simulink model "Proj_4"  (R2024a)
settings: Solver=VariableStepAuto  StartTime=0.0  StopTime=10.0  RelTol=1e-3
values from neighbouring files (symbols this model uses):
  rps2rpm = 60/(2*pi())    [wk3_init.m]
undefined symbols (not defined in the file or in its folder): batData, carData, motorData
libraries: slpidlib x1
settings Model: Creator=cbvaw  LastModifiedBy=stick
settings RTWCC: GPUComputeCapability=3.5

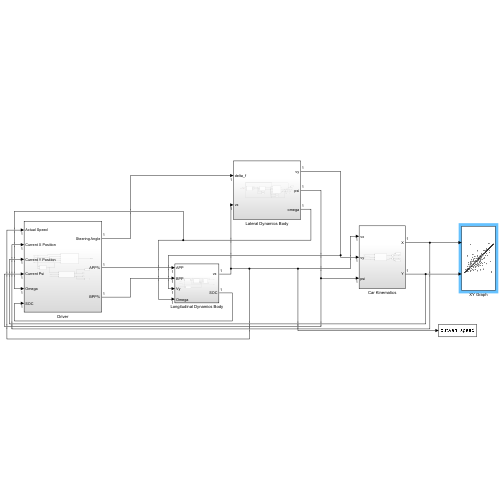
[thumbnail: Simulink's stored preview of the top-level diagram]
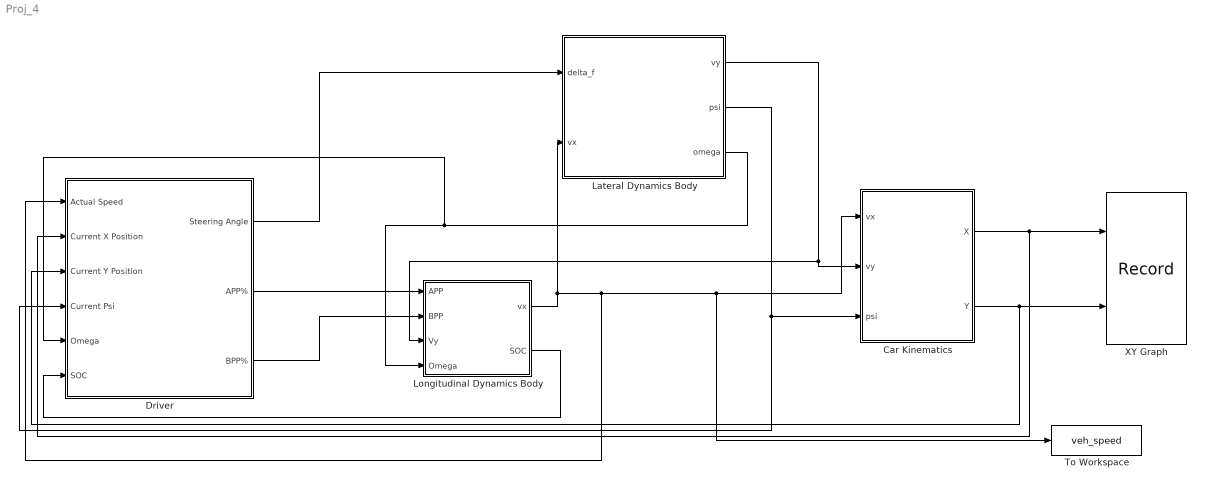
== system Proj_4 ==
  Car Kinematics : Subsystem
  Driver : Subsystem
  Lateral Dynamics Body : Subsystem
  Longitudinal Dynamics Body : Subsystem
  To Workspace : ToWorkspace  VariableName=veh_speed  SaveFormat=Structure With Time  SampleTime=-1
  XY Graph : Record  FileSettingsInternal="{\"entries\":[{\"content\":{\"excelSettings\":{\"content\":{},\"type\":\"Streamout.ExcelSettings\"}},\"type\":\"Streamout.FileSettingStorage\",\"uuid\":\"\"}],\"packageUris\":[\"http:\\/\\/schema.mathworks.com\\/mf0\\/streamout_blocks\\/R2020a\"],\"version\":\"1.0\"}"  Layout=[1 1]  SignalsInternal="{\"entries\":[{\"content\":{\"signals\":[{\"content\":{\"blockPath\":[],\"dimensions\":[1],\"domain\":\"\",\"lineColor\":\"#d95319\",\"plots\":[ 1 ],\"port\":1,\"signalID\":1,\"signalName\":\"CarKinematicsInertialFrame:1\"},\"type\":\"RecordBlkView.Signal\",\"uuid\":\"\"},{\"content\":{\"blockPath\":[],\"dimensions\":[1],\"domain\":\"\",\"lineColor\":\"#edb120\",\"plots\":[ 1 ],\"port\":2,\"signalID\":2,\"signalName\":\"CarKinematicsInertialFrame:2\"},\"type\":\"RecordBlkView.Signal\",\"uuid\":\"\"}]},\"type\":\"RecordBlkView.InputSignals\",\"uuid\":\"\"}],\"packageUris\":[\"http:\\/\\/schema.mathworks.com\\/mf0\\/streamout_blocks\\/R2020a\"],\"version\":\"1.0\"}"  VisualizationBindings="{\"xyplotplugin\":{\"info\":[{\"series\":[{\"bindingParametersList\":[{\"parameter\":\"X-Axis\",\"signalID\":1,\"signalName\":\"CarKinematicsInertialFrame:1\"},{\"parameter\":\"Y-Axis\",\"signalID\":2,\"signalName\":\"CarKinematicsInertialFrame:2\"}],\"seriesID\":0}],\"subplotID\":1}]}}"  CompatibilityTag=XY  st=-1
  wires:
  Car Kinematics/2(Y) -> Driver/3(Current Y Position), XY Graph/2
  Car Kinematics/1(X) -> Driver/2(Current X Position), XY Graph/1
  Lateral Dynamics Body/1(vy) -> Longitudinal Dynamics Body/3(Vy), Car Kinematics/2(vy)
  Lateral Dynamics Body/2(psi) -> Driver/4(Current Psi), Car Kinematics/3(psi)
  Longitudinal Dynamics Body/1("vx ") -> Driver/1(Actual Speed), To Workspace/1, Car Kinematics/1(vx), Lateral Dynamics Body/2(vx)
  Lateral Dynamics Body/3(omega) -> Driver/5(Omega), Longitudinal Dynamics Body/4(Omega)
  Driver/2(APP%) -> Longitudinal Dynamics Body/1(APP)
  Driver/3(BPP%) -> Longitudinal Dynamics Body/2(BPP)
  Driver/1(Steering Angle) -> Lateral Dynamics Body/1(delta_f)
  Longitudinal Dynamics Body/2(SOC) -> Driver/6(SOC)

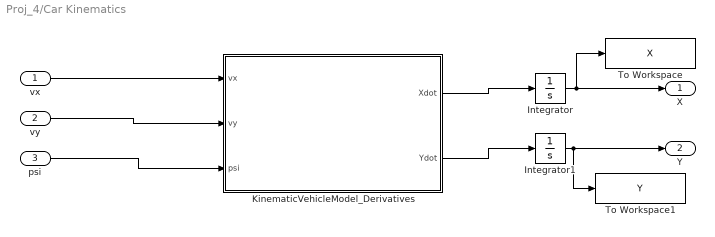
== system Proj_4/Car Kinematics ==
  vx : Inport
  vy : Inport  Port=2
  psi : Inport  Port=3
  Integrator : Integrator  InitialCondition=carData.init.X0
  Integrator1 : Integrator  InitialCondition=carData.init.Y0
  KinematicVehicleModel_Derivatives : MATLAB Function  TreatAsAtomicUnit=on
  To Workspace : ToWorkspace  VariableName=X  SaveFormat=Timeseries  SampleTime=-1
  To Workspace1 : ToWorkspace  VariableName=Y  SaveFormat=Timeseries  SampleTime=-1
  X : Outport
  Y : Outport  Port=2
  wires:
  Integrator1/1 -> To Workspace1/1, Y/1
  vy/1 -> KinematicVehicleModel_Derivatives/2(vy)
  vx/1 -> KinematicVehicleModel_Derivatives/1(vx)
  KinematicVehicleModel_Derivatives/2(Ydot) -> Integrator1/1
  psi/1 -> KinematicVehicleModel_Derivatives/3(psi)
  Integrator/1 -> To Workspace/1, X/1
  KinematicVehicleModel_Derivatives/1(Xdot) -> Integrator/1

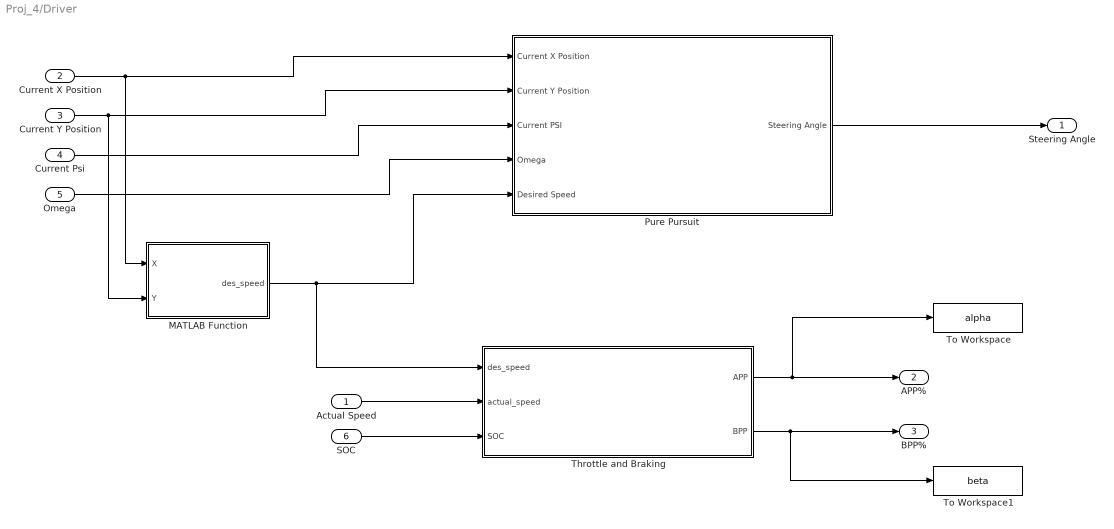
== system Proj_4/Driver ==
  Actual Speed : Inport
  Current X Position : Inport  Port=2
  Current Y Position : Inport  Port=3
  Current Psi : Inport  Port=4
  Omega : Inport  Port=5
  SOC : Inport  Port=6
  MATLAB Function : MATLAB Function  TreatAsAtomicUnit=on
  Pure Pursuit : Subsystem
  Throttle and Braking : Subsystem
  To Workspace : ToWorkspace  VariableName=alpha  SaveFormat=Timeseries  SampleTime=-1
  To Workspace1 : ToWorkspace  VariableName=beta  SaveFormat=Timeseries  SampleTime=-1
  Steering Angle : Outport
  APP% : Outport  Port=2
  BPP% : Outport  Port=3
  wires:
  Throttle and Braking/2(BPP) -> BPP%/1, To Workspace1/1
  Throttle and Braking/1(APP) -> APP%/1, To Workspace/1
  SOC/1 -> Throttle and Braking/3(SOC)
  Actual Speed/1 -> Throttle and Braking/2(actual_speed)
  Pure Pursuit/1(Steering Angle) -> Steering Angle/1
  MATLAB Function/1(des_speed) -> Pure Pursuit/5(Desired Speed), Throttle and Braking/1(des_speed)
  Omega/1 -> Pure Pursuit/4(Omega)
  Current Psi/1 -> Pure Pursuit/3(Current PSI)
  Current Y Position/1 -> MATLAB Function/2(Y), Pure Pursuit/2(Current Y Position)
  Current X Position/1 -> MATLAB Function/1(X), Pure Pursuit/1(Current X Position)

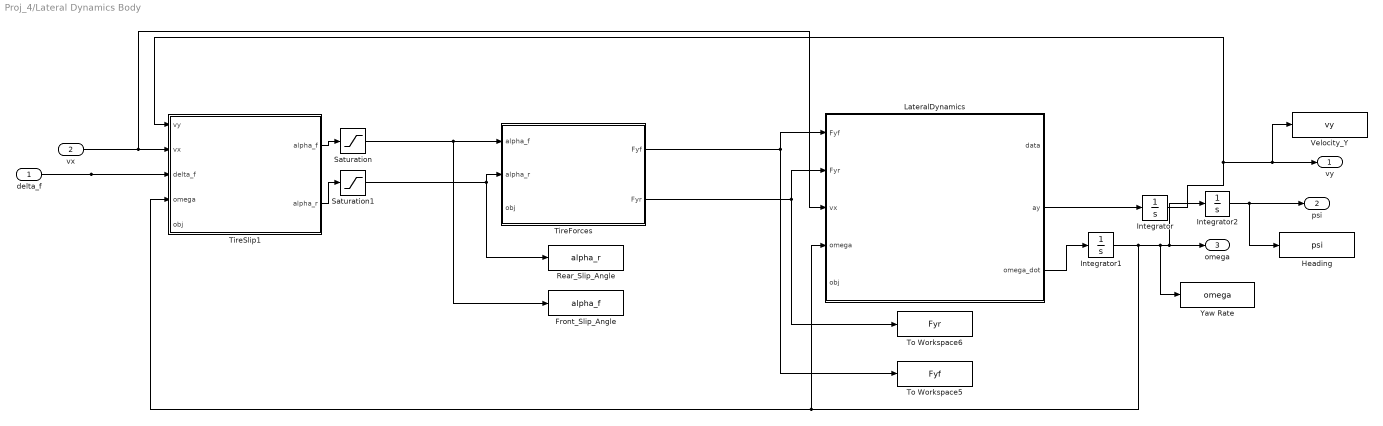
== system Proj_4/Lateral Dynamics Body ==
  delta_f : Inport
  vx : Inport  Port=2
  Front_Slip_Angle : ToWorkspace  VariableName=alpha_f  SaveFormat=Timeseries  SampleTime=-1
  Heading : ToWorkspace  VariableName=psi  SaveFormat=Timeseries  SampleTime=-1
  Integrator : Integrator  InitialCondition=carData.init.vy0
  Integrator1 : Integrator  InitialCondition=carData.init.omega0
  Integrator2 : Integrator  InitialCondition=carData.init.psi0  WrappedStateUpperValue=2*pi  WrappedStateLowerValue=0
  LateralDynamics : MATLAB Function  TreatAsAtomicUnit=on
  Rear_Slip_Angle : ToWorkspace  VariableName=alpha_r  SaveFormat=Timeseries  SampleTime=-1
  Saturation : Saturate  UpperLimit=carData.maxAlpha  LowerLimit=-carData.maxAlpha
  Saturation1 : Saturate  UpperLimit=carData.maxAlpha  LowerLimit=-carData.maxAlpha
  TireForces : MATLAB Function  TreatAsAtomicUnit=on
  TireSlip1 : MATLAB Function  TreatAsAtomicUnit=on
  To Workspace5 : ToWorkspace  VariableName=Fyf  SaveFormat=Timeseries  SampleTime=-1
  To Workspace6 : ToWorkspace  VariableName=Fyr  SaveFormat=Timeseries  SampleTime=-1
  Velocity_Y : ToWorkspace  VariableName=vy  SaveFormat=Timeseries  SampleTime=-1
  Yaw Rate : ToWorkspace  VariableName=omega  SaveFormat=Timeseries  SampleTime=-1
  vy : Outport
  psi : Outport  Port=2
  omega : Outport  Port=3
  wires:
  Integrator1/1 -> Integrator2/1, omega/1, Yaw Rate/1, LateralDynamics/4(omega), TireSlip1/4(omega)
  delta_f/1 -> TireSlip1/3(delta_f)
  Integrator/1 -> TireSlip1/1(vy), vy/1, Velocity_Y/1
  LateralDynamics/3(omega_dot) -> Integrator1/1
  Integrator2/1 -> Heading/1, psi/1
  LateralDynamics/2(ay) -> Integrator/1
  Saturation1/1 -> TireForces/2(alpha_r), Rear_Slip_Angle/1
  TireSlip1/1(alpha_f) -> Saturation/1
  vx/1 -> LateralDynamics/3(vx), TireSlip1/2(vx)
  TireForces/2(Fyr) -> LateralDynamics/2(Fyr), To Workspace6/1
  TireForces/1(Fyf) -> LateralDynamics/1(Fyf), To Workspace5/1
  Saturation/1 -> TireForces/1(alpha_f), Front_Slip_Angle/1
  TireSlip1/2(alpha_r) -> Saturation1/1

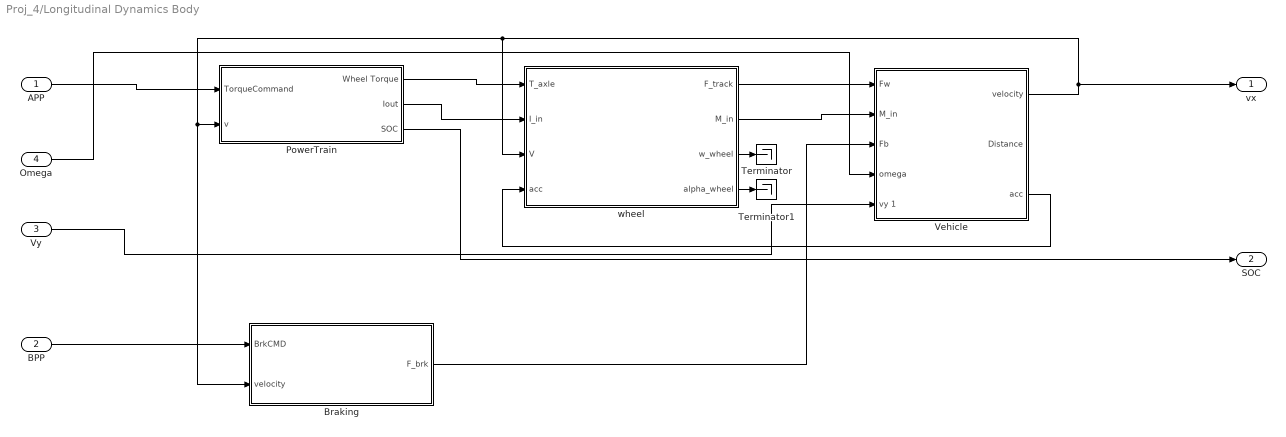
== system Proj_4/Longitudinal Dynamics Body ==
  APP : Inport
  BPP : Inport  Port=2
  Vy : Inport  Port=3
  Omega : Inport  Port=4
  Braking : Subsystem
  PowerTrain : Subsystem
  Terminator : Terminator
  Terminator1 : Terminator
  Vehicle : Subsystem
  "wheel " : Subsystem
  "vx " : Outport
  SOC : Outport  Port=2
  wires:
  PowerTrain/1(Wheel Torque) -> "wheel "/1(T_axle)
  PowerTrain/2(Iout) -> "wheel "/2(I_in)
  Braking/1("F_brk ") -> Vehicle/3("Fb ")
  "wheel "/2(M_in) -> Vehicle/2("M_in ")
  "wheel "/1(F_track) -> Vehicle/1("Fw ")
  Vehicle/1("velocity ") -> Braking/2("velocity "), PowerTrain/2(v), "wheel "/3(V), "vx "/1
  Vehicle/3(acc) -> "wheel "/4(acc)
  APP/1 -> PowerTrain/1(TorqueCommand)
  BPP/1 -> Braking/1("BrkCMD ")
  PowerTrain/3(SOC) -> SOC/1
  Vy/1 -> Vehicle/5(vy 1)
  Omega/1 -> Vehicle/4(omega)
  "wheel "/3(w_wheel) -> Terminator/1
  "wheel "/4(alpha_wheel) -> Terminator1/1

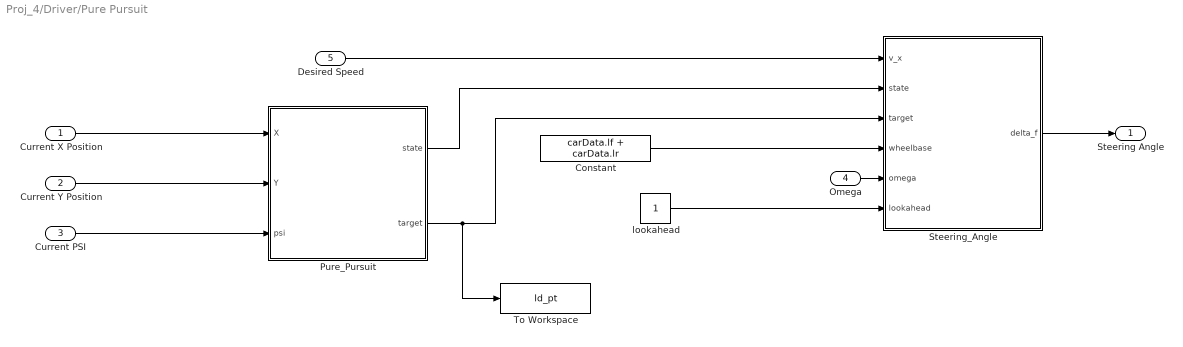
== system Proj_4/Driver/Pure Pursuit ==
  Current X Position : Inport
  Current Y Position : Inport  Port=2
  Current PSI : Inport  Port=3
  Omega : Inport  Port=4
  Desired Speed : Inport  Port=5
  Constant : Constant  Value=carData.lf + carData.lr
  Pure_Pursuit : MATLAB Function  TreatAsAtomicUnit=on
  Steering_Angle : MATLAB Function  TreatAsAtomicUnit=on
  To Workspace : ToWorkspace  VariableName=ld_pt  SaveFormat=Timeseries  SampleTime=-1
  lookahead : Constant
  Steering Angle : Outport
  wires:
  Constant/1 -> Steering_Angle/4(wheelbase)
  lookahead/1 -> Steering_Angle/6(lookahead)
  Steering_Angle/1(delta_f) -> Steering Angle/1
  Pure_Pursuit/2(target) -> Steering_Angle/3(target), To Workspace/1
  Omega/1 -> Steering_Angle/5(omega)
  Pure_Pursuit/1(state) -> Steering_Angle/2(state)
  Desired Speed/1 -> Steering_Angle/1(v_x)
  Current PSI/1 -> Pure_Pursuit/3(psi)
  Current Y Position/1 -> Pure_Pursuit/2(Y)
  Current X Position/1 -> Pure_Pursuit/1(X)

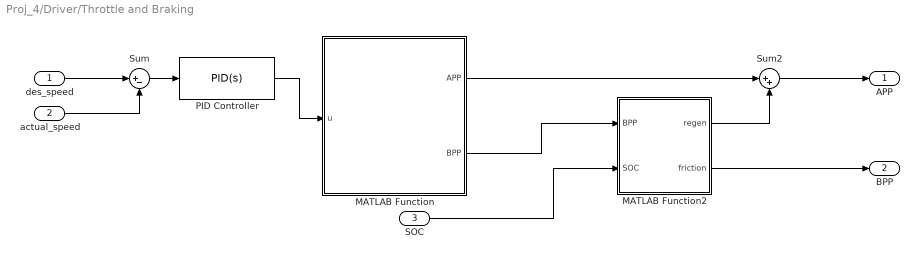
== system Proj_4/Driver/Throttle and Braking ==
  des_speed : Inport
  actual_speed : Inport  Port=2
  SOC : Inport  Port=3
  MATLAB Function : MATLAB Function  TreatAsAtomicUnit=on
  MATLAB Function2 : MATLAB Function  TreatAsAtomicUnit=on
  PID Controller : slpidlib/PID Controller  Controller=PID  Form=Parallel  TimeDomain=Continuous-time  UseExternalTs=off  SampleTime=-1  IntegratorMethod=Forward Euler  FilterMethod=Forward Euler  ControllerParametersSource=internal  P=.6  I=0  UseKiTs=off  D=.001  UseExternalDerivativeSource=off  N=100  UseFilter=on  TunerSelectOption=Transfer Function Based (PID Tuner App)  InitialConditionSource=internal  InitialConditionForIntegrator=0  InitialConditionForFilter=0  DifferentiatorICPrevScaledInput=0  ExternalReset=none  TrackingMode=off  Kt=1  LimitOutput=on  SatLimitsSource=internal  UpperSaturationLimit=1  LowerSaturationLimit=-1  LinearizeAsGain=off  AntiWindupMode=none  Kb=1  LimitIntegrator=off  UpperIntegratorSaturationLimit=inf  LowerIntegratorSaturationLimit=-inf  POutMin=[]  POutMax=[]  IOutMin=[]  IOutMax=[]  DOutMin=[]  DOutMax=[]  NOutMin=[]  NOutMax=[]  SumOutMin=[]  SumOutMax=[]  SaturationOutMin=[]  SaturationOutMax=[]  PParamMin=[]  PParamMax=[]  IParamMin=[]  IParamMax=[]  DParamMin=[]  DParamMax=[]  NParamMin=[]  NParamMax=[]  KbParamMin=[]  KbParamMax=[]  KtParamMin=[]  KtParamMax=[]  KbOutMin=[]  KbOutMax=[]  KtOutMin=[]  KtOutMax=[]  IntegratorOutMin=[]  IntegratorOutMax=[]  FilterOutMin=[]  FilterOutMax=[]  SumI1OutMin=[]  SumI1OutMax=[]  SumI2OutMin=[]  SumI2OutMax=[]  SumI3OutMin=[]  SumI3OutMax=[]  SumI4OutMin=[]  SumI4OutMax=[]  SumDOutMin=[]  SumDOutMax=[]  DifferentiatorOutMin=[]  DifferentiatorOutMax=[]  FilterDiffOutCoefMin=[]  FilterDiffOutCoefMax=[]  ReciprocalOutMin=[]  ReciprocalOutMax=[]  SumDenOutMin=[]  SumDenOutMax=[]  SumNumOutMin=[]  SumNumOutMax=[]  DivideOutMin=[]  DivideOutMax=[]  UdiffTsProdOutMin=[]  UdiffTsProdOutMax=[]  NTsProdOutMin=[]  NTsProdOutMax=[]  UintegralTsProdOutMin=[]  UintegralTsProdOutMax=[]  UngainTsProdOutMin=[]  UngainTsProdOutMax=[]  ClampingZeroOutDataTypeStr=Inherit: Inherit via back propagation  ClampingZeroOutMin=[]  ClampingZeroOutMax=[]  FilterDenConstantOutDataTypeStr=Inherit: Inherit via back propagation  FilterDenConstantOutMin=[]  FilterDenConstantOutMax=[]  PCopyOutDataTypeStr=Inherit: Inherit via back propagation  PCopyOutMin=[]  PCopyOutMax=[]  NCopyOutDataTypeStr=Inherit: Inherit via back propagation  NCopyOutMin=[]  NCopyOutMax=[]  IntegratorContinuousStateAttributes=''  IntegratorStateMustResolveToSignalObject=off  IntegratorRTWStateStorageClass=Auto  FilterContinuousStateAttributes=''  FilterStateMustResolveToSignalObject=off  FilterRTWStateStorageClass=Auto  ParallelPVariant=InternalParameters  IdealPVariant=Disabled  IVariant=InternalParameters  DVariant=InternalParameters  IntegratorVariant=Continuous  SatVariant=Enabled  AWVariant=Passthrough  PCopyVariant=Disabled  TRVariant=Disabled  FdbkBlocksVariant=Forward  IdealPFdbkVariant=Disabled  SatFdbkVariant=Disabled  DerivativeFilterVariant=ContFilter  NVariant=InternalParameters  NCopyVariant=Disabled  FilterICVariant=InternalICsFilter  IntegratorICVariant=InternalICs  ExternalResetVariant=Disabled  TRSumVariant=Passthrough  SumFdbkVariant=Disabled  SumVariant=Sum_PID  TsampFilterVariant=InternalTs  TsampNgainVariant=Passthrough  TsampIntegralVariant=Disabled_SignalSpec  ExternalSaturationOutDataTypeStr=Inherit: Same as second input  DerivativeSourceVariant=ErrorSignal
  Sum : Sum  Inputs=|+-
  Sum2 : Sum  Inputs=|++
  APP : Outport
  BPP : Outport  Port=2
  wires:
  MATLAB Function2/2(friction) -> BPP/1
  Sum2/1 -> APP/1
  MATLAB Function2/1(regen) -> Sum2/2
  PID Controller/1 -> MATLAB Function/1(u)
  Sum/1 -> PID Controller/1
  MATLAB Function/2(BPP) -> MATLAB Function2/1(BPP)
  MATLAB Function/1(APP) -> Sum2/1
  SOC/1 -> MATLAB Function2/2(SOC)
  actual_speed/1 -> Sum/2
  des_speed/1 -> Sum/1

== system Proj_4/Longitudinal Dynamics Body/Braking ==
  "BrkCMD " : Inport
  "velocity " : Inport  Port=2
  Gain1 : Gain  Gain=10000*carData.r
  MATLAB Function : MATLAB Function  TreatAsAtomicUnit=on
  "F_brk " : Outport  VectorParamsAs1DForOutWhenUnconnected=off
  wires:
  "BrkCMD "/1 -> Gain1/1
  Gain1/1 -> MATLAB Function/1(u)
  MATLAB Function/1(y) -> "F_brk "/1
  "velocity "/1 -> MATLAB Function/2(v)

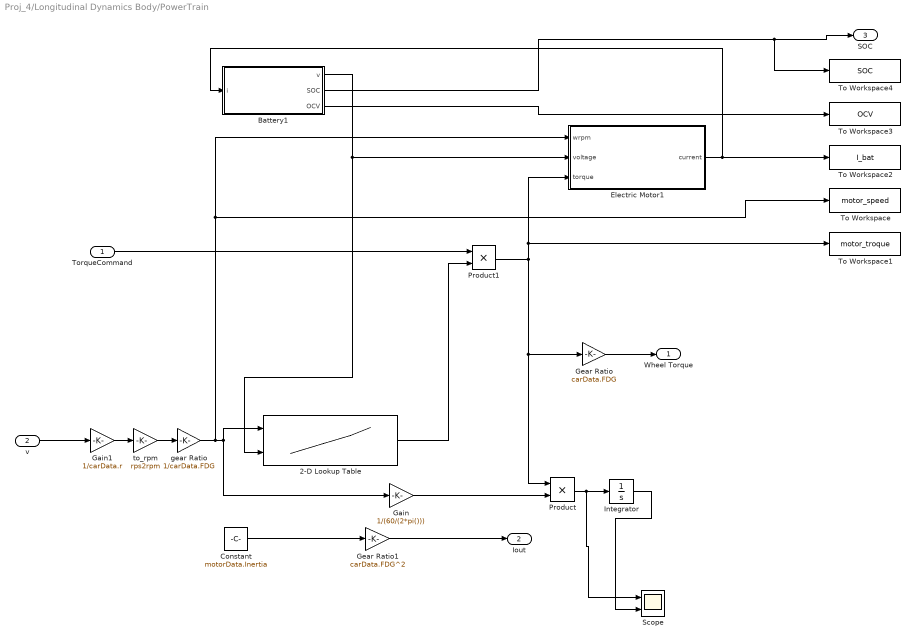
== system Proj_4/Longitudinal Dynamics Body/PowerTrain ==
  TorqueCommand : Inport
  v : Inport  Port=2
  2-D Lookup Table : Lookup_n-D  BreakpointsForDimension1=motorData.vbus  BreakpointsForDimension2=motorData.rpm  Table=motorData.maxtorque  InternalRulePriority=Speed  RndMeth=Simplest
      settings: InputPortMap=u0,u1
  Battery1 : Subsystem
  Constant : Constant  Value=motorData.Inertia
  Electric Motor1 : Subsystem
  Gain : Gain  Gain=1/(60/(2*pi()))
  Gain1 : Gain  Gain=1/carData.r
  Gear Ratio : Gain  Gain=carData.FDG
  Gear Ratio1 : Gain  Gain=carData.FDG^2
  Integrator : Integrator
  Product : Product
  Product1 : Product
  Scope : Scope  NumInputPorts=2
  To Workspace : ToWorkspace  VariableName=motor_speed  SaveFormat=Structure With Time  SampleTime=-1
  To Workspace1 : ToWorkspace  VariableName=motor_troque  SaveFormat=Structure With Time  SampleTime=-1
  To Workspace2 : ToWorkspace  VariableName=I_bat  SaveFormat=Structure With Time  SampleTime=-1
  To Workspace3 : ToWorkspace  VariableName=OCV  SaveFormat=Structure With Time  SampleTime=-1
  To Workspace4 : ToWorkspace  VariableName=SOC  SaveFormat=Structure With Time  SampleTime=-1
  gear Ratio : Gain  Gain=1/carData.FDG
  to_rpm : Gain  Gain=rps2rpm
  Wheel Torque : Outport
  Iout : Outport  Port=2
  SOC : Outport  Port=3
  wires:
  TorqueCommand/1 -> Product1/1
  Constant/1 -> Gear Ratio1/1
  v/1 -> Gain1/1
  Gain1/1 -> to_rpm/1
  2-D Lookup Table/1 -> Product1/2
  Product1/1 -> Product/1, Gear Ratio/1, Electric Motor1/3(torque), To Workspace1/1
  to_rpm/1 -> gear Ratio/1
  gear Ratio/1 -> Electric Motor1/1(wrpm), To Workspace/1, Gain/1, 2-D Lookup Table/1
  Gear Ratio/1 -> Wheel Torque/1
  Product/1 -> Scope/1, Integrator/1
  Integrator/1 -> Scope/2
  Gain/1 -> Product/2
  Battery1/1(v) -> 2-D Lookup Table/2, Electric Motor1/2(voltage)
  Electric Motor1/1(current) -> To Workspace2/1, Battery1/1(i)
  Gear Ratio1/1 -> Iout/1
  Battery1/2(SOC) -> To Workspace4/1, SOC/1
  Battery1/3(OCV) -> To Workspace3/1

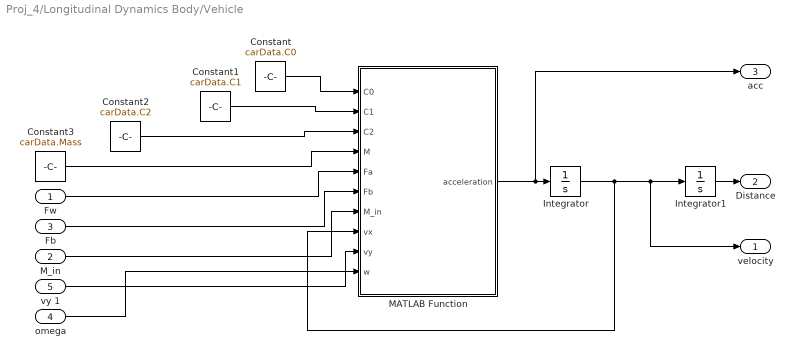
== system Proj_4/Longitudinal Dynamics Body/Vehicle ==
  "Fw " : Inport
  "M_in " : Inport  Port=2
  "Fb " : Inport  Port=3
  omega : Inport  Port=4
  vy 1 : Inport  Port=5
  Constant : Constant  Value=carData.C0
  Constant1 : Constant  Value=carData.C1
  Constant2 : Constant  Value=carData.C2
  Constant3 : Constant  Value=carData.Mass
  Integrator : Integrator  LimitOutput=on  LowerSaturationLimit=0
  Integrator1 : Integrator
  MATLAB Function : MATLAB Function  TreatAsAtomicUnit=on
  "velocity " : Outport  VectorParamsAs1DForOutWhenUnconnected=off
  "Distance " : Outport  Port=2  VectorParamsAs1DForOutWhenUnconnected=off
  acc : Outport  Port=3
  wires:
  Constant1/1 -> MATLAB Function/2(C1)
  Constant/1 -> MATLAB Function/1(C0)
  MATLAB Function/1(acceleration) -> acc/1, Integrator/1
  Constant2/1 -> MATLAB Function/3(C2)
  Constant3/1 -> MATLAB Function/4(M)
  "Fw "/1 -> MATLAB Function/5(Fa)
  "Fb "/1 -> MATLAB Function/6(Fb)
  Integrator/1 -> MATLAB Function/8(vx), "velocity "/1, Integrator1/1
  Integrator1/1 -> "Distance "/1
  "M_in "/1 -> MATLAB Function/7(M_in)
  omega/1 -> MATLAB Function/10(w)
  vy 1/1 -> MATLAB Function/9(vy)

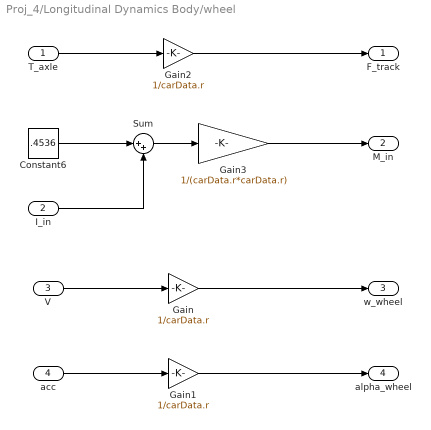
== system Proj_4/Longitudinal Dynamics Body/wheel  ==
  T_axle : Inport
  I_in : Inport  Port=2
  V : Inport  Port=3
  acc : Inport  Port=4
  Constant6 : Constant  Value=.4536
  Gain : Gain  Gain=1/carData.r
  Gain1 : Gain  Gain=1/carData.r
  Gain2 : Gain  Gain=1/carData.r
  Gain3 : Gain  Gain=1/(carData.r*carData.r)
  Sum : Sum  Inputs=|++
  F_track : Outport
  M_in : Outport  Port=2
  w_wheel : Outport  Port=3
  alpha_wheel : Outport  Port=4
  wires:
  Gain/1 -> w_wheel/1
  V/1 -> Gain/1
  acc/1 -> Gain1/1
  Gain1/1 -> alpha_wheel/1
  T_axle/1 -> Gain2/1
  Gain2/1 -> F_track/1
  Gain3/1 -> M_in/1
  Constant6/1 -> Sum/1
  I_in/1 -> Sum/2
  Sum/1 -> Gain3/1

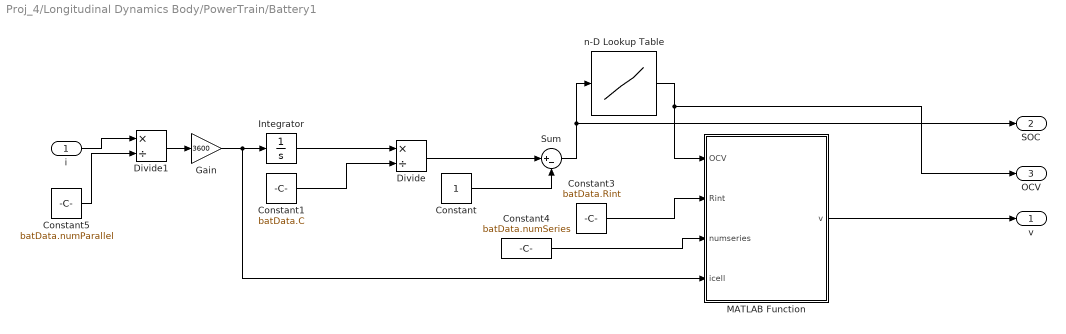
== system Proj_4/Longitudinal Dynamics Body/PowerTrain/Battery1 ==
  i : Inport
  Constant : Constant
  Constant1 : Constant  Value=batData.C
  Constant3 : Constant  Value=batData.Rint
  Constant4 : Constant  Value=batData.numSeries
  Constant5 : Constant  Value=batData.numParallel
  Divide : Product  Inputs=*/
  Divide1 : Product  Inputs=*/
  Gain : Gain  Gain=3600
  Integrator : Integrator
  MATLAB Function : MATLAB Function  TreatAsAtomicUnit=on
  Sum : Sum  Inputs=|+-
  n-D Lookup Table : Lookup_n-D  NumberOfTableDimensions=1  BreakpointsForDimension1=batData.SOC  BreakpointsForDimension3=[5, 7]  Table=batData.OCV  InternalRulePriority=Speed  RndMeth=Simplest
  v : Outport
  SOC : Outport  Port=2
  OCV : Outport  Port=3
  wires:
  Constant/1 -> Sum/2
  Integrator/1 -> Divide/1
  Divide/1 -> Sum/1
  Constant1/1 -> Divide/2
  MATLAB Function/1(v) -> v/1
  Constant4/1 -> MATLAB Function/3(numseries)
  Divide1/1 -> Gain/1
  Constant5/1 -> Divide1/2
  i/1 -> Divide1/1
  Constant3/1 -> MATLAB Function/2(Rint)
  Sum/1 -> SOC/1, n-D Lookup Table/1
  n-D Lookup Table/1 -> OCV/1, MATLAB Function/1(OCV)
  Gain/1 -> MATLAB Function/4(icell), Integrator/1

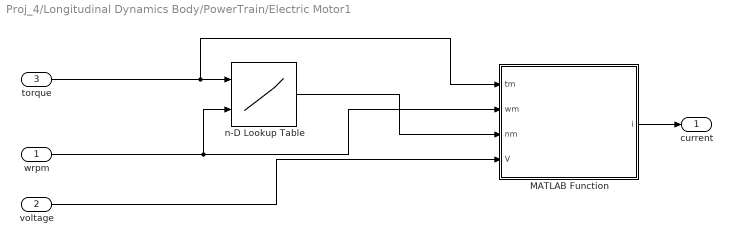
== system Proj_4/Longitudinal Dynamics Body/PowerTrain/Electric Motor1 ==
  wrpm : Inport
  voltage : Inport  Port=2
  torque : Inport  Port=3
  MATLAB Function : MATLAB Function  TreatAsAtomicUnit=on
  n-D Lookup Table : Lookup_n-D  BreakpointsForDimension1=motorData.eta_torque  BreakpointsForDimension2=motorData.eta_speed  BreakpointsForDimension3=[5, 7]  Table=motorData.eta_val  InternalRulePriority=Speed  RndMeth=Simplest
      settings: InputPortMap=u0,u1
  current : Outport
  wires:
  torque/1 -> MATLAB Function/1(tm), n-D Lookup Table/1
  wrpm/1 -> MATLAB Function/2(wm), n-D Lookup Table/2
  n-D Lookup Table/1 -> MATLAB Function/3(nm)
  MATLAB Function/1(i) -> current/1
  voltage/1 -> MATLAB Function/4(V)

== matlab function Proj_4/Driver/Pure Pursuit/Pure_Pursuit ==
  data: state output; target output; X input; Y input; psi input
function [state,target] = fcn(X,Y, psi)

dist = zeros(1, numel(waypoints_x));

for i = 1:numel(waypoints_x)
    dist(i) = sqrt((waypoints_x(i) - X)^2 + (waypoints_y(i) - Y)^2);

end

[~, index] = min(dist);

target_psi = atan2(waypoints_y(index) - Y, waypoints_x(index) - X);


state =[X,Y,psi];

target = [waypoints_x(index), waypoints_y(index), target_psi];

== matlab function Proj_4/Driver/Pure Pursuit/Steering_Angle ==
  data: v_x input; delta_f output; state input; target input; wheelbase input; omega input; lookahead input
function delta_f = fcn(v_x, state, target, wheelbase, omega, lookahead)

X = state(1);
Y = state(2);
psi = state(3);

target_X = target(1)
target_Y = target(2)
target_psi = target(3)

alpha = atan2(target_Y - Y, target_X - X) - psi;
psi_dot = (2 * wheelbase * sin(alpha)) / lookahead;
delta_f = atan(psi_dot);

== matlab function Proj_4/Driver/Throttle and Braking/MATLAB Function ==
  data: APP output; u input; BPP output
function [APP,BPP] = fcn(u)

if u>0
    APP=u;
    BPP=0;
elseif u<0
    APP=0;
    BPP=-u;
else
    APP=0;
    BPP=0;
end

== matlab function Proj_4/Driver/Throttle and Braking/MATLAB Function2 ==
  data: BPP input; regen output; friction output; SOC input
function [regen, friction] = fcn(BPP,SOC)

if actual_speed < 5
    friction = BPP;
    regen = 0;

elseif actual_speed >= 5 && actual_speed <= 25
    friction = BPP * ((100 - 4.75 * (actual_speed - 5)) / 100);
    regen = (1 - ((100 - 4.75 * (actual_speed - 5)) / 100)) * BPP;

else
    friction = 0.05 * BPP;
    regen = 0.95 * BPP;

end

if SOC >= 95
    friction = BPP;
    regen = 0;
end

== matlab function Proj_4/Lateral Dynamics Body/TireSlip1 ==
  data: vy input; alpha_f output; vx input; delta_f input; omega input; obj input; alpha_r output
function [alpha_f, alpha_r] = fnc(vy, vx, delta_f, omega, obj)

    if abs(vx) > obj.vx_threshold1
        alpha_f = delta_f - (vy + omega * obj.lf) / vx;
        alpha_r = - (vy - omega * obj.lr) / vx;
    else
        alpha_f = 0;
        alpha_r = 0;
    end

end

== matlab function Proj_4/Lateral Dynamics Body/LateralDynamics ==
  data: data output; Fyf input; ay output; Fyr input; vx input; omega input; obj input; omega_dot output
function [data, ay, omega_dot] = fcn(Fyf, Fyr, vx, omega, obj)

    Fy = Fyf + Fyr;
    ay = Fy / obj.Mass - omega * vx;

    M = Fyf * obj.lf - Fyr * obj.lr;
    omega_dot = M / obj.Inertia;

end

== matlab function Proj_4/Longitudinal Dynamics Body/PowerTrain/Electric Motor1/MATLAB Function ==
  data: tm input; i output; wm input; nm input; V input
function i = fcn(tm,wm,nm,V)

i = (tm*wm*(nm^((tm*wm)/(abs(tm*wm)+0.001)))) / V;

== matlab function Proj_4/Car Kinematics/KinematicVehicleModel_Derivatives ==
  data: vx input; Xdot output; vy input; psi input; Ydot output
function [Xdot, Ydot] = fcn(vx, vy, psi)
    temp = TF(psi) * [vx;vy];
    Xdot = temp(1);
    Ydot = temp(2);
end

function y = TF(psi)
    y = [cos(psi), -sin(psi); sin(psi), cos(psi)];
end

== matlab function Proj_4/Longitudinal Dynamics Body/Braking/MATLAB Function ==
  data: u input; y output; v input
function y = fcn(u,v)
y = u * v/(abs(v)+0.001);

== matlab function Proj_4/Longitudinal Dynamics Body/PowerTrain/Battery1/MATLAB Function ==
  data: v output; OCV input; Rint input; numseries input; icell input
function v = fcn(OCV, Rint, numseries, icell)

v = numseries * (OCV - Rint * icell) ;

== matlab function Proj_4/Lateral Dynamics Body/TireForces ==
  data: alpha_f input; Fyf output; alpha_r input; obj input; Fyr output
function [Fyf, Fyr] = fcn(alpha_f, alpha_r, obj)

    Fyf = min(obj.Fyfmax, obj.Calpha_f * alpha_f);
    Fyr = min(obj.Fyrmax, obj.Calpha_r * alpha_r);

end

== matlab function Proj_4/Longitudinal Dynamics Body/Vehicle/MATLAB Function ==
  data: C0 input; acceleration output; C1 input; C2 input; M input; Fa input; Fb input; M_in input; vx input; vy input; w input
function acceleration   = vehicle(C0,C1,C2,M,Fa,Fb,M_in, vx, vy, w)

acceleration = (((Fa-Fb))-(C0+ C1*vx + C2*(vx)^2 + 9.8*M + vy*w))/(M+M_in);

== matlab function Proj_4/Driver/MATLAB Function ==
  data: X input; des_speed output; Y input
function des_speed = fcn(X,Y)

des_speed = ;
